simulink model "OutputEvents"  (R2024a)
settings: Solver=FixedStepDiscrete  StartTime=0.0  StopTime=10.0  RelTol=1e-3
settings Model: Creator=VICTUS  LastModifiedBy=VICTUS

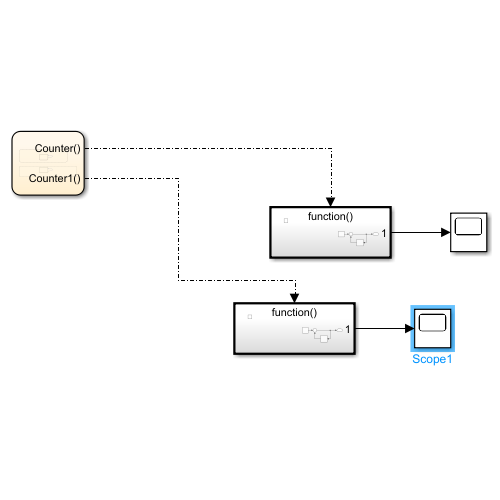
[thumbnail: Simulink's stored preview of the top-level diagram]
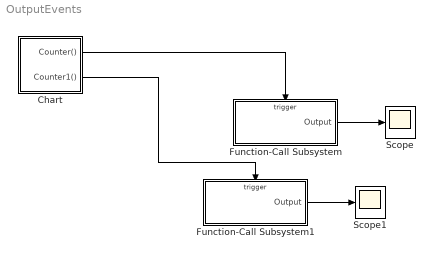
== system OutputEvents ==
  Chart : Stateflow chart  TreatAsAtomicUnit=on
  Function-Call Subsystem : Subsystem  TreatAsAtomicUnit=on
  Function-Call Subsystem1 : Subsystem  TreatAsAtomicUnit=on
  Scope : Scope
  Scope1 : Scope
  wires:
  Chart/1(Counter()) -> Function-Call Subsystem/Trigger
  Function-Call Subsystem/1(Output) -> Scope/1
  Function-Call Subsystem1/1(Output) -> Scope1/1
  Chart/2(Counter1()) -> Function-Call Subsystem1/Trigger

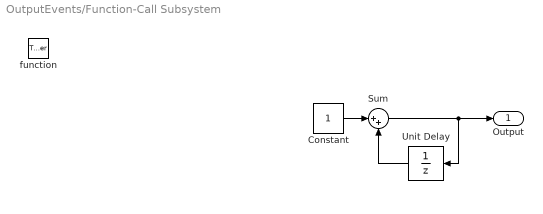
== system OutputEvents/Function-Call Subsystem ==
  function : TriggerPort  TriggerType=function-call  VariantControl=(inherit)
  Constant : Constant
  Sum : Sum  Inputs=|++
  Unit Delay : UnitDelay  SampleTime=-1  HasFrameUpgradeWarning=on
  Output : Outport
  wires:
  Sum/1 -> Output/1, Unit Delay/1
  Constant/1 -> Sum/1
  Unit Delay/1 -> Sum/2

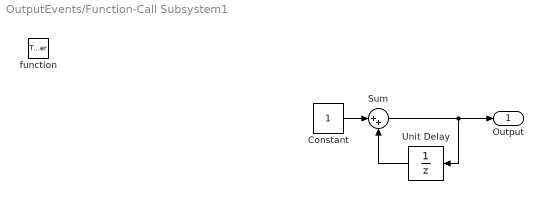
== system OutputEvents/Function-Call Subsystem1 ==
  function : TriggerPort  TriggerType=function-call  VariantControl=(inherit)
  Constant : Constant
  Sum : Sum  Inputs=|++
  Unit Delay : UnitDelay  SampleTime=-1  HasFrameUpgradeWarning=on
  Output : Outport
  wires:
  Unit Delay/1 -> Sum/2
  Constant/1 -> Sum/1
  Sum/1 -> Unit Delay/1, Output/1

== stateflow chart OutputEvents/Chart ==
  state S3 [parallel]
    settings: executionOrder=1
    state S1
    S1 -> S1 : after(1,sec)/{Counter}
  state S4 [parallel]
    settings: executionOrder=2
    state S2
    S2 -> S2 : after(0.5,sec)/{Counter1}
  events: Counter output FUNCTION_CALL_EVENT; Counter1 output FUNCTION_CALL_EVENT
